simulink model "Connect_OPCUA"  (R2022a)
settings: Solver=VariableStepAuto  StartTime=0.0  StopTime=10.0  RelTol=1e-3
settings Model: Creator=intel  LastModifiedBy=Aalae

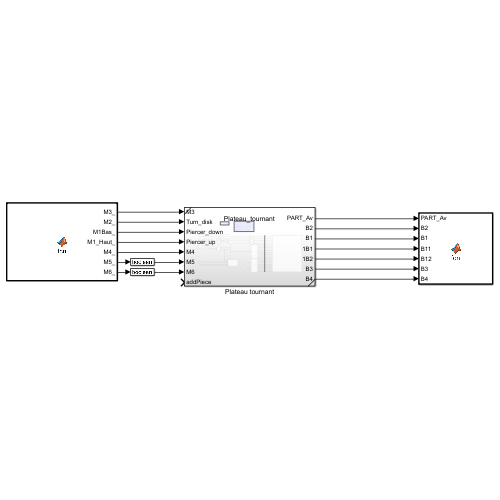
[thumbnail: Simulink's stored preview of the top-level diagram]
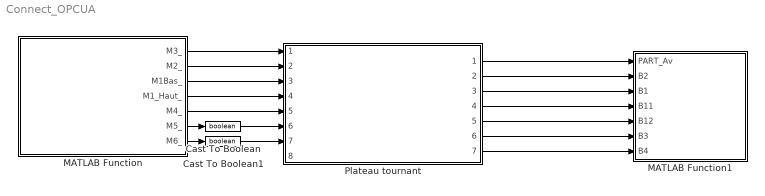
== system Connect_OPCUA ==
  Cast To Boolean : DataTypeConversion  OutDataTypeStr=boolean  SaturateOnIntegerOverflow=off  RndMeth=Floor
  Cast To Boolean1 : DataTypeConversion  OutDataTypeStr=boolean  SaturateOnIntegerOverflow=off  RndMeth=Floor
  MATLAB Function : MATLAB Function  TreatAsAtomicUnit=on
  MATLAB Function1 : MATLAB Function  TreatAsAtomicUnit=on
  Plateau tournant : Subsystem  ReferencedSubsystem=Plateau_tournant
  wires:
  MATLAB Function/1(M3_) -> Plateau tournant/1
  MATLAB Function/2(M2_) -> Plateau tournant/2
  MATLAB Function/3(M1Bas_) -> Plateau tournant/3
  MATLAB Function/4(M1_Haut_) -> Plateau tournant/4
  MATLAB Function/5(M4_) -> Plateau tournant/5
  Plateau tournant/1 -> MATLAB Function1/1(PART_Av)
  Plateau tournant/2 -> MATLAB Function1/2(B2)
  Plateau tournant/3 -> MATLAB Function1/3(B1)
  Plateau tournant/4 -> MATLAB Function1/4(B11)
  Plateau tournant/5 -> MATLAB Function1/5(B12)
  Plateau tournant/6 -> MATLAB Function1/6(B3)
  Plateau tournant/7 -> MATLAB Function1/7(B4)
  MATLAB Function/6(M5_) -> Cast To Boolean/1
  MATLAB Function/7(M6_) -> Cast To Boolean1/1
  Cast To Boolean1/1 -> Plateau tournant/7
  Cast To Boolean/1 -> Plateau tournant/6

== matlab function Connect_OPCUA/MATLAB Function ==
  data: M3_ output; M2_ output; M1Bas_ output; M1_Haut_ output; M4_ output; M5_ output; M6_ output
function [M3_,M2_,M1Bas_,M1_Haut_,M4_,M5_,M6_] = fcn()

coder.extrinsic('Read_DTOPC_Func'); 

M3_ = false;
M2_ = false;
M1Bas_ = false;
M1_Haut_ = false;
M4_ = false;
M5_ = false;
M6_ = false;

[M3_,M2_,M1Bas_,M1_Haut_,M4_,M5_,M6_] = Read_DTOPC_Func();

== matlab function Connect_OPCUA/MATLAB Function1 ==
  data: PART_Av input; B2 input; B1 input; B11 input; B12 input; B3 input; B4 input
function fcn(PART_Av, B2, B1, B11, B12, B3, B4)

coder.extrinsic('Write_DTOPC_Func'); 

Write_DTOPC_Func([PART_Av, B2, B1, B11, B12, B3, B4]);
